simulink model "offlineProcessing"  (Simulink 8.3)
settings: Solver=ode45  StartTime=0.0  StopTime=10  RelTol=1e-3
undefined symbols (not defined in the file or in its folder): alphaMS, FS, magnitude, numSamplesPer20msFrame, psdMinBuf
libraries: dspsigops x3, dspxfrm3 x2, dspstat3 x2, dspmathops x1, dspsrcs4 x1, dspsnks4 x1
settings Model: Creator=Abhi  LastModifiedBy=Abhi
settings DataIOCC: SignalLoggingSaveFormat=Dataset
settings DebuggingCC: UnderspecifiedInitializationDetection=Simplified  SolverPrmCheckMsg=none  StateNameClashWarn=none
settings GRTTargetCC: CombineOutputUpdateFcns=on  GRTInterface=off

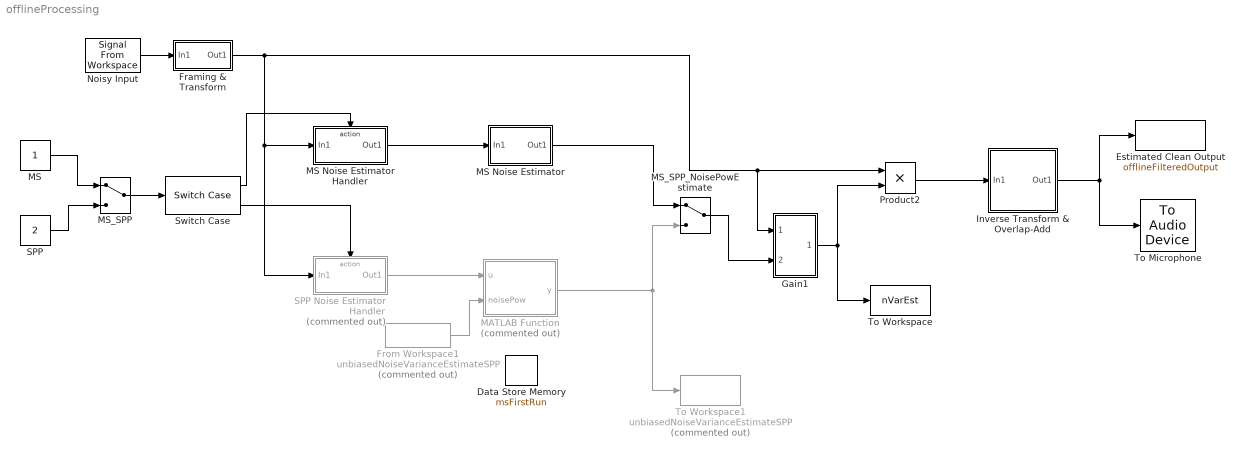
== system offlineProcessing ==
  Data Store Memory : DataStoreMemory  DataStoreName=msFirstRun  ReadBeforeWriteMsg=warning  WriteAfterWriteMsg=warning  WriteAfterReadMsg=warning  InitialValue=1  OutDataTypeStr=boolean
  Estimated Clean Output : ToWorkspace  VariableName=offlineFilteredOutput  SaveFormat=Structure  SampleTime=-1
      settings: Save2DSignal=2-D array (concatenate along first dimension)
  Framing & Transform : Subsystem
  From Workspace1 : FromWorkspace  Commented=on  VariableName=unbiasedNoiseVarianceEstimateSPP  SampleTime=0
  Gain1 : Subsystem
  Inverse Transform & Overlap-Add : Subsystem
  MATLAB Function : MATLAB Function  Commented=on  TreatAsAtomicUnit=on
  MS : Constant
  MS Noise Estimator : Subsystem
  MS Noise Estimator Handler : Subsystem  TreatAsAtomicUnit=on
  MS_SPP : ManualSwitch
  MS_SPP_NoisePowEstimate : ManualSwitch
  Noisy Input : dspsrcs4/Signal From Workspace  X=noisyInput  Ts=1/FS  nsamps=numSamplesPer20msFrame  OutputAfterFinalValue=Setting to zero  ignoreOrWarnInputAndFrameLengths=off
  Product2 : Product
  SPP : Constant  Value=2
  SPP Noise Estimator Handler : Subsystem  Commented=on  TreatAsAtomicUnit=on
  Switch Case : SwitchCase  CaseConditions={1,2}  ShowDefaultCase=off
  To Microphone : dspsnks4/To Audio Device  deviceName=Default  inheritSampleRate=on  sampleRate=44100  deviceDatatype=Determine from input data type  autoBufferSize=on  bufferSize=4096  queueDuration=1.0  defaultOutputChannelMapping=on  outputChannelMapping=1:2
  To Workspace : ToWorkspace  VariableName=nVarEst  SaveFormat=Timeseries  SampleTime=-1
  To Workspace1 : ToWorkspace  Commented=on  VariableName=unbiasedNoiseVarianceEstimateSPP  SaveFormat=Timeseries  SampleTime=-1
  wires:
  Noisy Input/1 -> Framing & Transform/1(In1)
  Inverse Transform & Overlap-Add/1(Out1) -> Estimated Clean Output/1, To Microphone/1
  Switch Case/1 -> MS Noise Estimator Handler/Action
  Switch Case/2 -> SPP Noise Estimator Handler/Action
  Framing & Transform/1(Out1) -> Gain1/1(In1), Product2/1, SPP Noise Estimator Handler/1(In1), MS Noise Estimator Handler/1(In1)
  SPP Noise Estimator Handler/1(Out1) -> MATLAB Function/1(u)
  MATLAB Function/1(y) -> To Workspace1/1, MS_SPP_NoisePowEstimate/2
  From Workspace1/1 -> MATLAB Function/2(noisePow)
  Gain1/1(Out1) -> Product2/2, To Workspace/1
  MS_SPP/1 -> Switch Case/1
  MS/1 -> MS_SPP/1
  SPP/1 -> MS_SPP/2
  Product2/1 -> Inverse Transform & Overlap-Add/1(In1)
  MS Noise Estimator/1(Out1) -> MS_SPP_NoisePowEstimate/1
  MS Noise Estimator Handler/1(Out1) -> MS Noise Estimator/1(In1)
  MS_SPP_NoisePowEstimate/1 -> Gain1/2(In2)

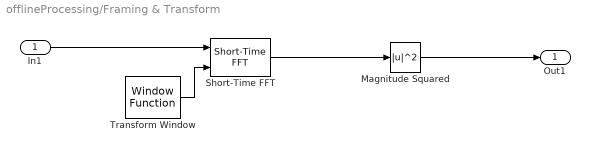
== system offlineProcessing/Framing & Transform ==
  In1 : Inport
  Magnitude Squared : Math  Operator=magnitude^2  SaturateOnIntegerOverflow=on
  Short-Time FFT : dspxfrm3/Short-Time FFT  W=numSamplesPer20msFrame  OvLap=overlapSamples  M=numSamplesPer20msFrame  TreatMby1Signals=One channel
  Transform Window : dspsigops/Window Function  winmode=Generate window  wintype=Hanning  sampmode=Discrete  samptime=1  N=numSamplesPer20msFrame  Rs=50  beta=10  winsamp=Symmetric  UserWindow=hamming  OptParams=off  UserParams={'symmetric'}  RowConvenienceOn=on  dataType=double  isSigned=on  wordLen=16  udDataType=sfix(16)  fracBitsMode=Best precision  numFracBits=15  roundingMode=Floor  overflowMode=off  numSidelobes=4  sidelobeLevel=-30
  Out1 : Outport
  wires:
  Short-Time FFT/1 -> Magnitude Squared/1
  Transform Window/1 -> Short-Time FFT/2
  In1/1 -> Short-Time FFT/1
  Magnitude Squared/1 -> Out1/1

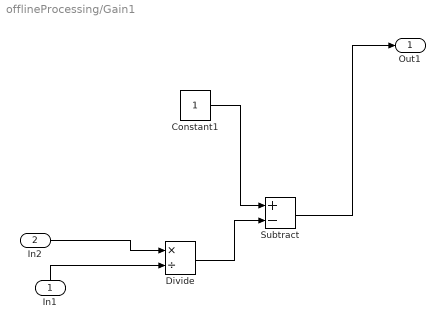
== system offlineProcessing/Gain1 ==
  In1 : Inport
  In2 : Inport  Port=2
  Constant1 : Constant
  Divide : Product  Inputs=*/
  Subtract : Sum  Inputs=+-
  Out1 : Outport
  wires:
  Subtract/1 -> Out1/1
  Divide/1 -> Subtract/2
  Constant1/1 -> Subtract/1
  In1/1 -> Divide/2
  In2/1 -> Divide/1

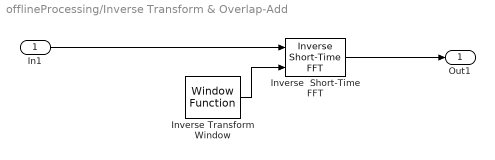
== system offlineProcessing/Inverse Transform & Overlap-Add ==
  In1 : Inport
  Inverse Transform Window : dspsigops/Window Function  winmode=Generate window  wintype=Hanning  sampmode=Discrete  samptime=1  N=numSamplesPer20msFrame  Rs=50  beta=10  winsamp=Symmetric  UserWindow=hamming  OptParams=off  UserParams={'symmetric'}  RowConvenienceOn=on  dataType=double  isSigned=on  wordLen=16  udDataType=sfix(16)  fracBitsMode=Best precision  numFracBits=15  roundingMode=Floor  overflowMode=off  numSidelobes=4  sidelobeLevel=-30
  Inverse  Short-Time FFT : dspxfrm3/Inverse  Short-Time FFT  W=numSamplesPer20msFrame  OvLap=overlapSamples  OutFrameSize=numSamplesPer20msFrame  InConjSymm=on  DoAssert=off  Tol=1e-4
  Out1 : Outport
  wires:
  Inverse  Short-Time FFT/1 -> Out1/1
  Inverse Transform Window/1 -> Inverse  Short-Time FFT/2
  In1/1 -> Inverse  Short-Time FFT/1

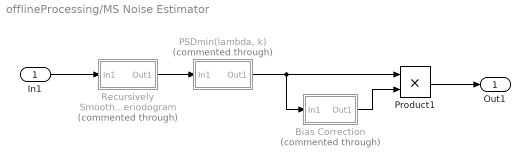
== system offlineProcessing/MS Noise Estimator ==
  In1 : Inport
  Bias Correction : Subsystem  Commented=through
  "PSDmin(lambda, k)" : Subsystem  Commented=through
  Product1 : Product
  Recursively Smoothed Periodogram : Subsystem  Commented=through
  Out1 : Outport
  wires:
  "PSDmin(lambda, k)"/1(Out1) -> Bias Correction/1(In1), Product1/1
  In1/1 -> Recursively Smoothed Periodogram/1(In1)
  Bias Correction/1(Out1) -> Product1/2
  Product1/1 -> Out1/1
  Recursively Smoothed Periodogram/1(Out1) -> "PSDmin(lambda, k)"/1(In1)

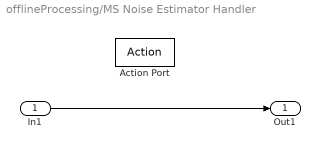
== system offlineProcessing/MS Noise Estimator Handler ==
  In1 : Inport
  Action Port : ActionPort  ActionType=case
  Out1 : Outport
  wires:
  In1/1 -> Out1/1

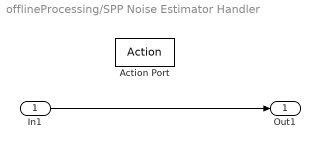
== system offlineProcessing/SPP Noise Estimator Handler ==
  In1 : Inport
  Action Port : ActionPort  ActionType=case
  Out1 : Outport
  wires:
  In1/1 -> Out1/1

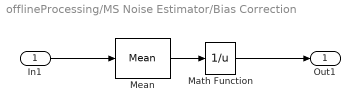
== system offlineProcessing/MS Noise Estimator/Bias Correction ==
  In1 : Inport
  Math Function : Math  Operator=reciprocal  SampleTime=1  SaturateOnIntegerOverflow=on
  Mean : dspstat3/Mean  run=on  reset_popup=None  InputProcessing=Columns as channels (frame based)  directionMode=Each column  dimension=1  treatSBRowAsCol=on  roiEnable=off  roiType=Rectangles  roiPortion=Entire ROI  roiOutput=Individual statistics for each ROI  roiFlag=off  outputDataTypeStr=Inherit: Same as accumulator  outputLastDataTypeStr=Inherit: Same as accumulator  outputMin=[]  outputMax=[]  roundingMode=Floor  overflowMode=off
  Out1 : Outport
  wires:
  Math Function/1 -> Out1/1
  Mean/1 -> Math Function/1
  In1/1 -> Mean/1

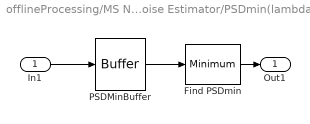
== system offlineProcessing/MS Noise Estimator/PSDmin(lambda, k) ==
  In1 : Inport
  Find PSDmin : dspstat3/Minimum  fcn=Value  reset=None  InputProcessing=Columns as channels (frame based)  indexBase=One  operateOver=Each column  Dimension=1  colComp=on  operation=minimum  roiEnable=off  roiType=Rectangles  roiPortion=Entire ROI  roiOutput=Individual statistics for each ROI  roiFlag=off  roundingMode=Floor  overflowMode=off
  PSDMinBuffer : Buffer  N=psdMinBuf  V=psdMinBuf-1  TreatMby1Signals=One channel
  Out1 : Outport
  wires:
  PSDMinBuffer/1 -> Find PSDmin/1
  In1/1 -> PSDMinBuffer/1
  Find PSDmin/1 -> Out1/1

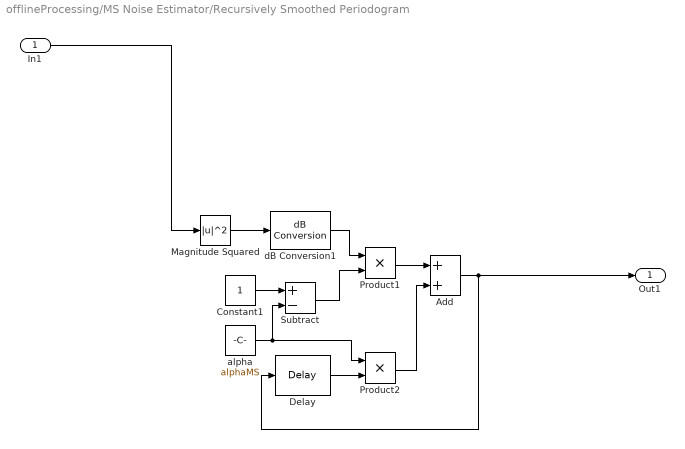
== system offlineProcessing/MS Noise Estimator/Recursively Smoothed Periodogram ==
  In1 : Inport
  Add : Sum
  Constant1 : Constant
  Delay : dspsigops/Delay  InputProcessing=Columns as channels (frame based)  dly_unit=Frames  delay=1  ic_detail=off  dif_ic_for_ch=off  dif_ic_for_dly=off  ic=0  reset_popup=None
  Magnitude Squared : Math  Operator=magnitude^2  SampleTime=1  SaturateOnIntegerOverflow=on
  Product1 : Product
  Product2 : Product  SampleTime=1
  Subtract : Sum  Inputs=+-
  alpha : Constant  Value=alphaMS
  dB Conversion1 : dspmathops/dB Conversion  dBtype=dB  intype=Power  R=1  fuzz=on
  Out1 : Outport
  wires:
  Product2/1 -> Add/2
  In1/1 -> Magnitude Squared/1
  Add/1 -> Out1/1, Delay/1
  alpha/1 -> Product2/1, Subtract/2
  Product1/1 -> Add/1
  Constant1/1 -> Subtract/1
  dB Conversion1/1 -> Product1/1
  Delay/1 -> Product2/2
  Subtract/1 -> Product1/2
  Magnitude Squared/1 -> dB Conversion1/1

== matlab function MATLAB Function ==
  data: u input double; y output double; noisePow input double; msFirstRun data_store_memory double
function y = fcn(u, noisePow)

global msFirstRun;

%% initialize
if msFirstRun == true
    %noisePow = init_noise_tracker_ideal_vad(u,frLen,frLen,fShift, anWin); % This function computes the initial noise PSD estimate. It is assumed that the first 5 time-frames are noise-only.
    y = zeros(size(u));
    msFirstRun = false;
    return;
end

%
PH1mean  = 0.5;
alphaPH1mean = 0.9;
alphaPSD = 0.8;

%constants for a posteriori SPP
q          = 0.5; % a priori probability of speech presence:
priorFact  = q./(1-q); % EQN (15) ???
% Fixing 15dB as the a priori SNR -> PAGE 6 Right (bottom)
xiOptDb    = 15; % optimal fixed a priori SNR for SPP estimation
xiOpt      = 10.^(xiOptDb./10);
logGLRFact = log(1./(1+xiOpt));
GLRexp     = xiOpt./(1+xiOpt);

% for indFr = 1:nFrames
%     indices       = (indFr-1)*fShift+1:(indFr-1)*fShift+frLen;
%     noisy_frame   = anWin.*noisy(indices);
%     noisyDftFrame = fft(noisy_frame,frLen); %512
%     noisyDftFrame = noisyDftFrame(1:frLen/2+1); %256
	
%     noisyPer = noisyDftFrame.*conj(noisyDftFrame); % <-(1)
    noisyPer = u.*conj(u); % <-(1)
    snrPost1 =  noisyPer./(noisePow);% a posteriori SNR based on old noise power estimate


    %% noise power estimation
	GLR     = priorFact .* exp(min(logGLRFact + GLRexp.*snrPost1,200));
	PH1     = GLR./(1+GLR); % a posteriori speech presence probability

	PH1mean  = alphaPH1mean * PH1mean + (1-alphaPH1mean) * PH1; % EQN (23)
	stuckInd = PH1mean > 0.99;                                  
	PH1(stuckInd) = min(PH1(stuckInd),0.99);                    % EQN (24)
	estimate =  PH1 .* noisePow + (1-PH1) .* noisyPer ; % noisyPer is obtained from DFT of windowed data over frame length -> (1) EQN (22)
	noisePow = alphaPSD *noisePow+(1-alphaPSD)*estimate;                                                                        % EQN (7)
        
% 	noisePowMat(:,indFr) = noisePow;
    y = noisePow;
% end
return





%%%%%%%%%%%%%%%%%%%%%%%%%%%%%%%%%%%%%%%%%%%%%%%%%%%%%%%%%%%%%%%%%%%%%%%%%%%%%%%%%%%%%%%


function   noise_psd_init =init_noise_tracker_ideal_vad(noisy,fr_size,fft_size,hop,sq_hann_window)
%%%%%%%%%%%%%%%%%%%%%%%%%%%%%%%%%%%%%%
%%%%This m-file computes an initial noise PSD estimate by means of a
%%%%Bartlett estimate.
%%%%Input parameters:   noisy:          noisy signal
%%%%                    fr_size:        frame size
%%%%                    fft_size:       fft size
%%%%                    hop:            hop size of frame
%%%%                    sq_hann_window: analysis window
%%%%Output parameters:  noise_psd_init: initial noise PSD estimate
%%%%
%%%%%%%%%%%%%%%%%%%%%%%%%%%%%%%%%%%%%%%%%%
%%%%%%%%%%%%%%%%%%%%%%Author: Richard C. Hendriks, 15/4/2010
%%%%%%%%%%%%%%%%%%%%%%%
%%%%%%%%%%%%%%%%%%%%%
 noisy_dft_frame_matrix = zeros(fft_size, 5);
for I=1:5
    noisy_frame=sq_hann_window.*noisy((I-1)*hop+1:(I-1)*hop+fr_size);
    noisy_dft_frame_matrix(:,I)=fft(noisy_frame,fft_size);
end
noise_psd_init=mean(abs(noisy_dft_frame_matrix(1:fr_size/2+1,1:end)).^2,2);%%%compute the initialisation of the noise tracking algorithms.
return
